simulink model "cpp_sim"  (R2025b)
settings: Solver=FixedStepAuto  StartTime=0.0  StopTime=56.7  FixedStep=0.1  RelTol=1e-3
undefined symbols (not defined in the file): cpp_angVel, cpp_linVel
libraries: matrix_library x1
settings Model: Creator=Riley Martin  LastModifiedBy=Riley Martin

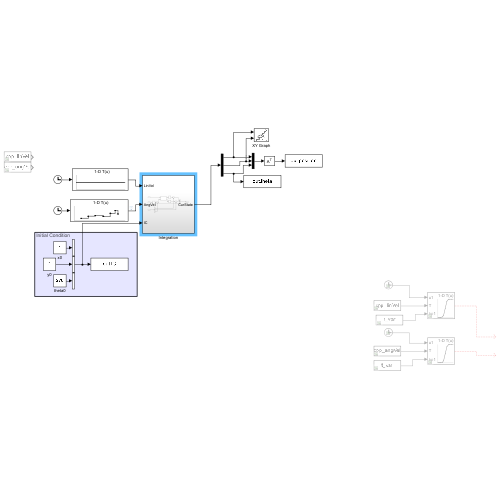
[thumbnail: Simulink's stored preview of the top-level diagram]
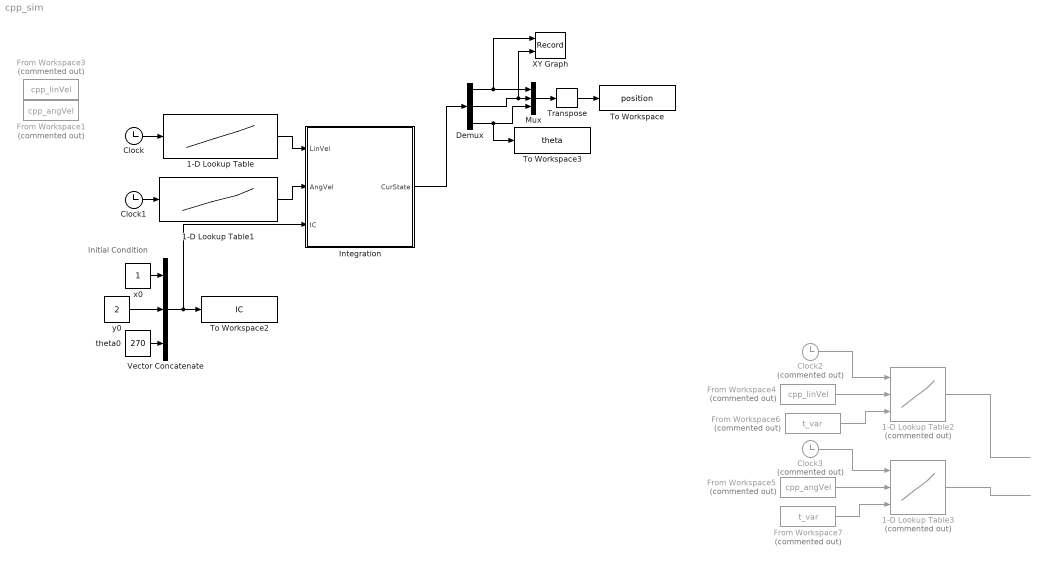
== system cpp_sim ==
  note: Initial Condition
  1-D Lookup Table : Lookup_n-D  NumberOfTableDimensions=1  BreakpointsForDimension1=cpp_linVel(:,1)  Table=cpp_linVel(:,2)  InternalRulePriority=Speed  RndMeth=Simplest
  1-D Lookup Table1 : Lookup_n-D  NumberOfTableDimensions=1  BreakpointsForDimension1=cpp_angVel(:,1)  Table=cpp_angVel(:,2)  InterpMethod=Nearest  InternalRulePriority=Speed  RndMeth=Simplest
  1-D Lookup Table2 : Lookup_n-D  Commented=on  NumberOfTableDimensions=1  BreakpointsForDimension1Source=Input port  BreakpointsForDimension1=[-5:5]  TableSource=Input port  Table=tanh([-5:5])  InternalRulePriority=Speed  RndMeth=Simplest
      settings: InputPortMap=u0,p221,p5
  1-D Lookup Table3 : Lookup_n-D  Commented=on  NumberOfTableDimensions=1  BreakpointsForDimension1Source=Input port  BreakpointsForDimension1=[-5:5]  TableSource=Input port  Table=tanh([-5:5])  InternalRulePriority=Speed  RndMeth=Simplest
      settings: InputPortMap=u0,p221,p5
  Clock : Clock
  Clock1 : Clock
  Clock2 : Clock  Commented=on
  Clock3 : Clock  Commented=on
  Demux : Demux  Outputs=3
  From Workspace1 : FromWorkspace  Commented=on  VariableName=cpp_angVel
  From Workspace3 : FromWorkspace  Commented=on  VariableName=cpp_linVel
  From Workspace4 : FromWorkspace  Commented=on  VariableName=cpp_linVel  OutDataTypeStr=double
  From Workspace5 : FromWorkspace  Commented=on  VariableName=cpp_angVel
  From Workspace6 : FromWorkspace  Commented=on  VariableName=t_var  OutDataTypeStr=double
  From Workspace7 : FromWorkspace  Commented=on  VariableName=t_var  OutDataTypeStr=double
  Integration : Subsystem
  Mux : Mux  Inputs=3
  To Workspace : ToWorkspace  VariableName=position  SaveFormat=Timeseries  SampleTime=-1
  To Workspace2 : ToWorkspace  VariableName=IC  SampleTime=-1
      settings: Save2DSignal=2-D array (concatenate along first dimension)
  To Workspace3 : ToWorkspace  VariableName=theta  SaveFormat=Timeseries  SampleTime=-1
  Transpose : matrix_library/Transpose
  Vector Concatenate : Concatenate  NumInputs=3
  XY Graph : Record  NumPorts=2.0  FileSettingsInternal="{\"entries\":[{\"content\":{\"excelSettings\":{\"content\":{},\"type\":\"Streamout.ExcelSettings\"},\"parquetSettings\":{\"content\":{},\"type\":\"Streamout.ParquetSettings\"}},\"type\":\"Streamout.FileSettingStorage\",\"uuid\":\"\"}],\"packageUris\":[\"http:\\/\\/schema.mathworks.com\\/mf0\\/streamout_blocks\\/R2020a\"],\"version\":\"1.0\"}"  FrameSettings=[0, 0]  Layout=[1 1]  SignalsInternal="{\"entries\":[{\"content\":{\"signals\":[{\"content\":{\"blockPath\":[],\"dimensions\":[1],\"domain\":\"\",\"lineColor\":\"#a2142f\",\"plots\":[ 1 ],\"port\":1,\"sid\":[\"\"],\"signalID\":1,\"signalName\":\"Demux:1\"},\"type\":\"RecordBlkView.Signal\",\"uuid\":\"\"},{\"content\":{\"blockPath\":[],\"dimensions\":[1],\"domain\":\"\",\"lineColor\":\"#139fff\",\"plots\":[ 1 ],\"port\":2,\"sid\":[\"\"],\"signalID\":2,\"signalName\":\"Demux:2\"},\"type\":\"RecordBlkView.Signal\",\"uuid\":\"\"}]},\"type\":\"RecordBlkView.InputSignals\",\"uuid\":\"\"}],\"packageUris\":[\"http:\\/\\/schema.mathworks.com\\/mf0\\/streamout_blocks\\/R2020a\"],\"version\":\"1.0\"}"  VisualizationBindings="{\"xyplotplugin\":{\"info\":[{\"series\":[],\"subplotID\":1}]}}"  CompatibilityTag=XY
  theta0 : Constant  Value=270
  x0 : Constant
  y0 : Constant  Value=2
  wires:
  y0/1 -> Vector Concatenate/2
  Vector Concatenate/1 -> Integration/3(IC), To Workspace2/1
  x0/1 -> Vector Concatenate/1
  theta0/1 -> Vector Concatenate/3
  Demux/2 -> XY Graph/2, Mux/2
  Demux/3 -> Mux/3, To Workspace3/1
  Demux/1 -> XY Graph/1, Mux/1
  Integration/1(CurState) -> Demux/1
  Mux/1 -> Transpose/1
  Transpose/1 -> To Workspace/1
  Clock/1 -> 1-D Lookup Table/1
  1-D Lookup Table/1 -> Integration/1(LinVel)
  Clock1/1 -> 1-D Lookup Table1/1
  1-D Lookup Table1/1 -> Integration/2(AngVel)
  1-D Lookup Table3/1 -> ?
  Clock2/1 -> 1-D Lookup Table2/1
  From Workspace7/1 -> 1-D Lookup Table3/3
  Clock3/1 -> 1-D Lookup Table3/1
  From Workspace5/1 -> 1-D Lookup Table3/2
  From Workspace6/1 -> 1-D Lookup Table2/3
  1-D Lookup Table2/1 -> ?
  From Workspace4/1 -> 1-D Lookup Table2/2

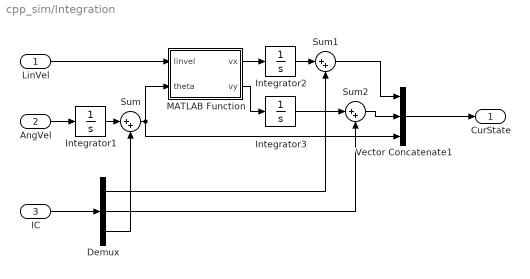
== system cpp_sim/Integration ==
  LinVel : Inport
  AngVel : Inport  Port=2
  IC : Inport  Port=3
  Demux : Demux  Outputs=3
  Integrator1 : Integrator
  Integrator2 : Integrator
  Integrator3 : Integrator
  MATLAB Function : MATLAB Function  TreatAsAtomicUnit=on
  Sum : Sum  Inputs=|++
  Sum1 : Sum  Inputs=|++
  Sum2 : Sum  Inputs=|++
  Vector Concatenate1 : Concatenate  NumInputs=3
  CurState : Outport
  wires:
  MATLAB Function/1(vx) -> Integrator2/1
  MATLAB Function/2(vy) -> Integrator3/1
  AngVel/1 -> Integrator1/1
  LinVel/1 -> MATLAB Function/1(linvel)
  Vector Concatenate1/1 -> CurState/1
  Integrator1/1 -> Sum/1
  Demux/3 -> Sum/2
  Integrator2/1 -> Sum1/1
  Demux/1 -> Sum1/2
  Demux/2 -> Sum2/2
  Integrator3/1 -> Sum2/1
  Sum2/1 -> Vector Concatenate1/2
  Sum1/1 -> Vector Concatenate1/1
  IC/1 -> Demux/1
  Sum/1 -> MATLAB Function/2(theta), Vector Concatenate1/3

== matlab function cpp_sim/Integration/MATLAB Function ==
  data: linvel input; vx output; theta input; vy output
function [vx,vy] = fcn(linvel,theta)
    vx = linvel*cos(theta);
    vy = linvel*sin(theta);
end
